simulink model "Boost_Simplified_Model_to_begin"  (R2024b)
settings: Solver=VariableStepAuto  StartTime=0.0  StopTime=10.0  MaxStep=1e-4  RelTol=1e-9
values from neighbouring files (symbols this model uses):
  C = .07e-3    (= 7e-05)    [Parameters.m]    (also in prelim.m)
  D_ss = 0.6    [Parameters.m]    (also in prelim.m)
  iL_ss = VO_ss/(R*(1-D_ss))    (= 5.625)    [prelim.m]
  L = .3e-3    (= 0.0003)    [Parameters.m]    (also in prelim.m)
  VO_ss = V_in/(1-D_ss)    (= 22.5)    [prelim.m]
undefined symbols (not defined in the file or in its folder): K_ex
settings Model: Creator=jkord  LastModifiedBy=Αναστασία Λίβα

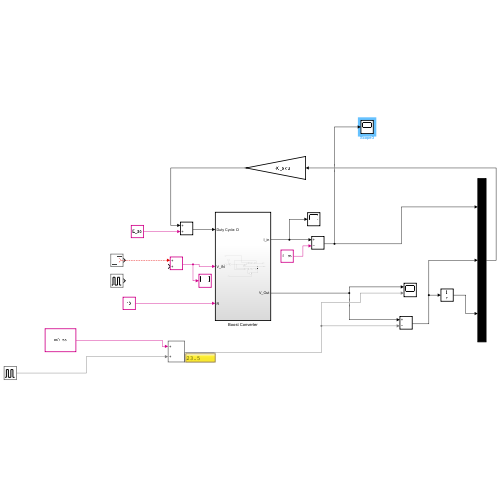
[thumbnail: Simulink's stored preview of the top-level diagram]
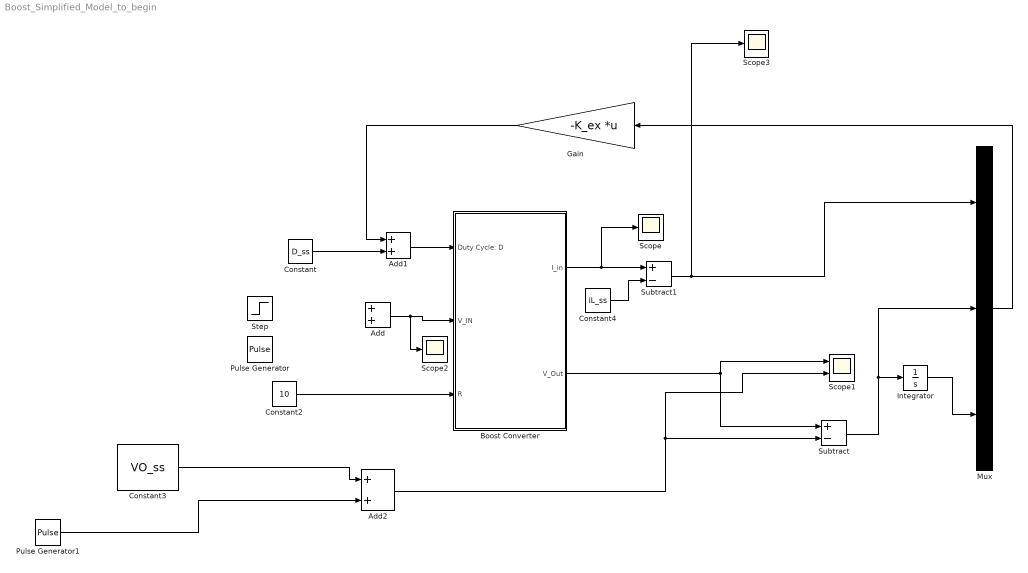
== system Boost_Simplified_Model_to_begin ==
  Add : Sum
  Add1 : Sum
  Add2 : Sum
  Boost Converter : Subsystem
  Constant : Constant  Value=D_ss
  Constant2 : Constant  Value=10
  Constant3 : Constant  Value=VO_ss
  Constant4 : Constant  Value=iL_ss
  Gain : Gain  Gain=-K_ex  Multiplication=Matrix(K*u)
  Integrator : Integrator
  Mux : Mux  Inputs=3
  Pulse Generator : DiscretePulseGenerator  PulseType=Time based  Amplitude=12  Period=0.5  PulseWidth=30
  Pulse Generator1 : DiscretePulseGenerator  PulseType=Time based  Period=0.5  PulseWidth=30
  Scope : Scope
  Scope1 : Scope  NumInputPorts=2
  Scope2 : Scope
  Scope3 : Scope
  Step : Step  SampleTime=0
  Subtract : Sum  Inputs=+-
  Subtract1 : Sum  Inputs=+-
  wires:
  Constant2/1 -> Boost Converter/3(R)
  Boost Converter/2(V_Out) -> Subtract/1, Scope1/1
  Boost Converter/1(I_in) -> Subtract1/1, Scope/1
  ? -> Add/1
  Add/1 -> Scope2/1, Boost Converter/2(V_IN)
  Constant/1 -> Add1/2
  Add2/1 -> Scope1/2, Subtract/2
  Constant3/1 -> Add2/1
  Pulse Generator1/1 -> Add2/2
  Subtract1/1 -> Scope3/1, Mux/1
  Subtract/1 -> Mux/2, Integrator/1
  Integrator/1 -> Mux/3
  Constant4/1 -> Subtract1/2
  Add1/1 -> Boost Converter/1(Duty Cycle: D)
  Mux/1 -> Gain/1
  Gain/1 -> Add1/1

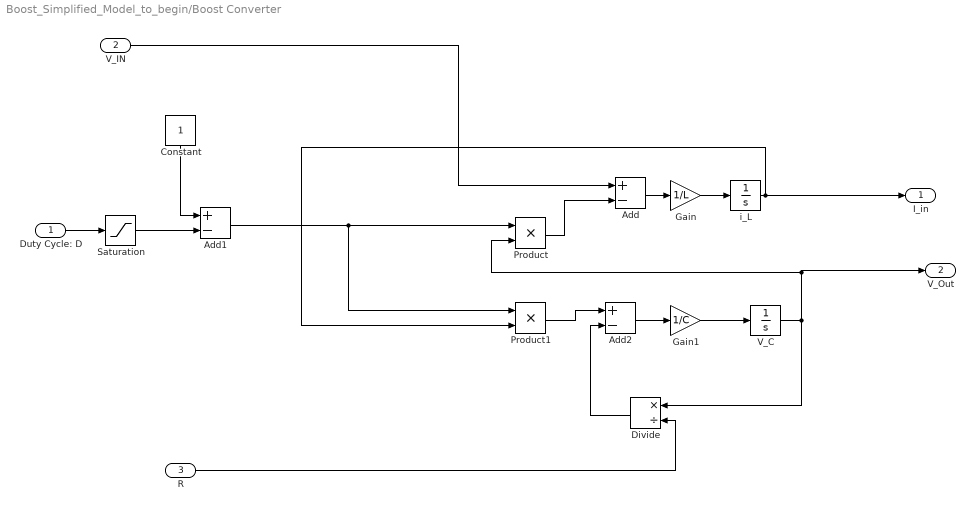
== system Boost_Simplified_Model_to_begin/Boost Converter ==
  Duty Cycle: D : Inport
  V_IN : Inport  Port=2
  R : Inport  Port=3
  Add : Sum  Inputs=+-
  Add1 : Sum  Inputs=+-
  Add2 : Sum  Inputs=+-
  Constant : Constant
  Divide : Product  Inputs=*/
  Gain : Gain  Gain=1/L
  Gain1 : Gain  Gain=1/C
  Product : Product
  Product1 : Product
  Saturation : Saturate  UpperLimit=0.9  LowerLimit=0.1
  V_C : Integrator  InitialCondition=10
  i_L : Integrator  InitialCondition=2
  I_in : Outport
  V_Out : Outport  Port=2
  wires:
  Product/1 -> Add/2
  i_L/1 -> I_in/1, Product1/2
  Gain1/1 -> V_C/1
  V_IN/1 -> Add/1
  Gain/1 -> i_L/1
  V_C/1 -> Divide/1, V_Out/1, Product/2
  Add/1 -> Gain/1
  Product1/1 -> Add2/1
  Add2/1 -> Gain1/1
  Divide/1 -> Add2/2
  R/1 -> Divide/2
  Duty Cycle: D/1 -> Saturation/1
  Saturation/1 -> Add1/2
  Constant/1 -> Add1/1
  Add1/1 -> Product1/1, Product/1
